simulink model "Simulink"  (R2023a)
settings: Solver=VariableStepAuto  StartTime=0.0  StopTime=10.0  RelTol=1e-3
values from neighbouring files (symbols this model uses):
  A = [1 -2 ... (first row only)    [hw4_2d_gulumjanli.m]    (also in hw4_p2a_gulumjanli.m; hw4_p2b_gulumjanli.m; hw4_p3a_gulumjanli.m = [  0         1       0; hw4_p3b_gulumjanli.m = [  0         1       0)
  B = [4.1; 2]    [hw4_2d_gulumjanli.m]    (also in hw4_p2a_gulumjanli.m = [2; hw4_p2b_gulumjanli.m = [2; 2]; hw4_p3a_gulumjanli.m = [0; hw4_p3b_gulumjanli.m = [0)
  C = [-1 1]    [hw4_2d_gulumjanli.m]    (also in hw4_p2a_gulumjanli.m; hw4_p2b_gulumjanli.m; hw4_p3a_gulumjanli.m = [1 0 0]; hw4_p3b_gulumjanli.m = [1 0 0])
  K = place(A, B, desired_poles)    [hw4_p3b_gulumjanli.m]    (also in hw4_p3c_gulumjanli.m)
settings Model: Creator=zqcsu656  LastModifiedBy=zqcsu656

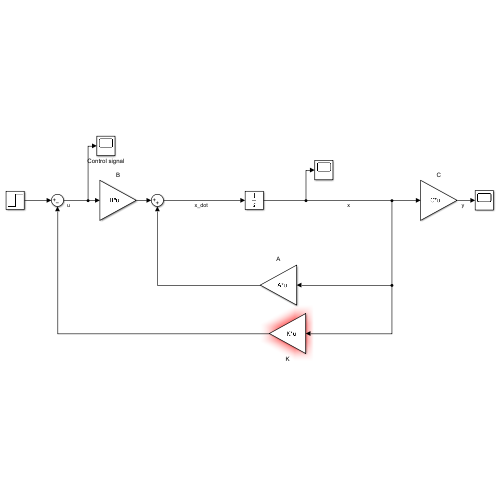
[thumbnail: Simulink's stored preview of the top-level diagram]
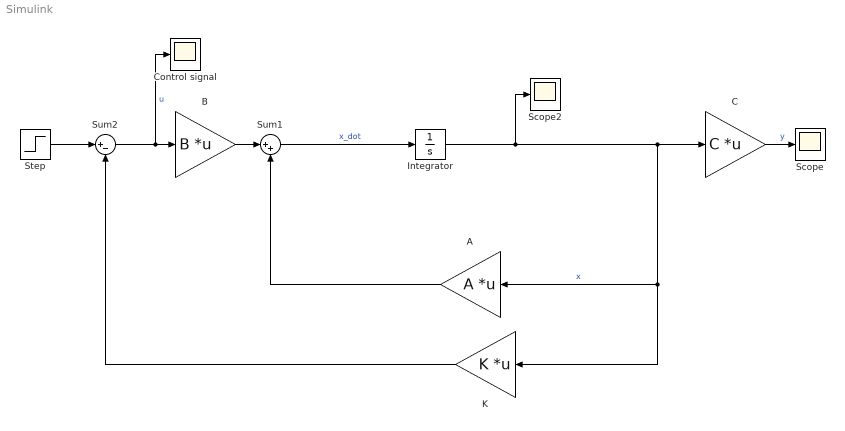
== system Simulink ==
  A : Gain  Gain=A  Multiplication=Matrix(K*u)
  B : Gain  Gain=B  Multiplication=Matrix(K*u)
  C : Gain  Gain=C  Multiplication=Matrix(K*u)
  Control signal : Scope
  Integrator : Integrator
  K : Gain  Gain=K  Multiplication=Matrix(K*u)
  Scope : Scope
  Scope2 : Scope
  Step : Step  Time=0  SampleTime=0
  Sum1 : Sum  Inputs=|++
  Sum2 : Sum  Inputs=|+-
  wires:
  Sum2/1 -> Control signal/1, B/1  "u"
  Sum1/1 -> Integrator/1  "x_dot"
  Integrator/1 -> Scope2/1, K/1, A/1, C/1  "x"
  A/1 -> Sum1/2
  B/1 -> Sum1/1
  C/1 -> Scope/1  "y"
  Step/1 -> Sum2/1
  K/1 -> Sum2/2
